simulink model "Disturb_test"  (R2019a)
settings: Solver=VariableStepAuto  StartTime=0.0  StopTime=10.0  RelTol=1e-3
settings Model: Creator=mario  LastModifiedBy=mario

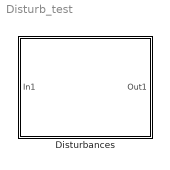
== system Disturb_test ==
  "Disturbances " : Subsystem

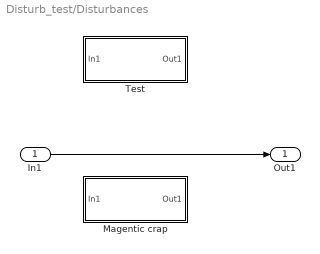
== system Disturb_test/Disturbances  ==
  In1 : Inport
  Magentic crap : Subsystem
  "Test " : Subsystem
  Out1 : Outport
  wires:
  In1/1 -> Out1/1

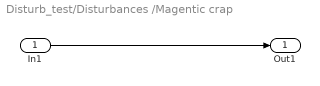
== system Disturb_test/Disturbances /Magentic crap ==
  In1 : Inport
  Out1 : Outport
  wires:
  In1/1 -> Out1/1

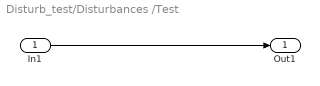
== system Disturb_test/Disturbances /Test  ==
  In1 : Inport
  Out1 : Outport
  wires:
  In1/1 -> Out1/1
